simulink model "BoostPFC_ELL437"  (R2022a)
settings: Solver=ode4  StartTime=0.0  StopTime=0.7  FixedStep=1e-7  RelTol=1e-3
undefined symbols (not defined in the file): C, fac, fs_PFC, Gci_inf, Gcv_inf, H, kx, L, R, Rs, vcontrol, Vm, Vref, wLi, wLv
libraries: spsDiodeLib x5, spsSeriesRLCBranchLib x3, spsVoltageMeasurementLib x2, spsACVoltageSourceLib x1, spsCurrentMeasurementLib x1, spsMosfetLib x1, simulink x1, spspowerguiLib x1
settings Model: Creator=Aditya Bhalotia  LastModifiedBy=Aditya Bhalotia
settings DataIOCC: ReturnWorkspaceOutputs=off

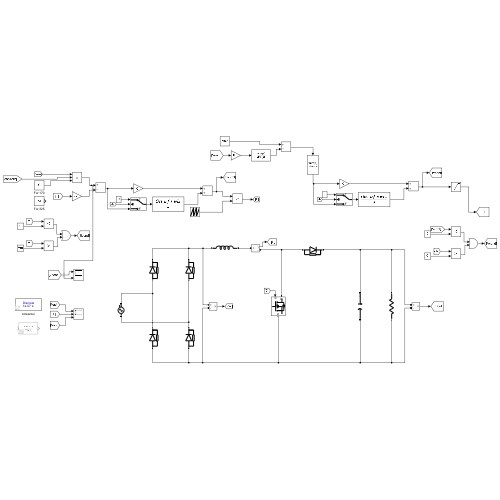
[thumbnail: Simulink's stored preview of the top-level diagram]
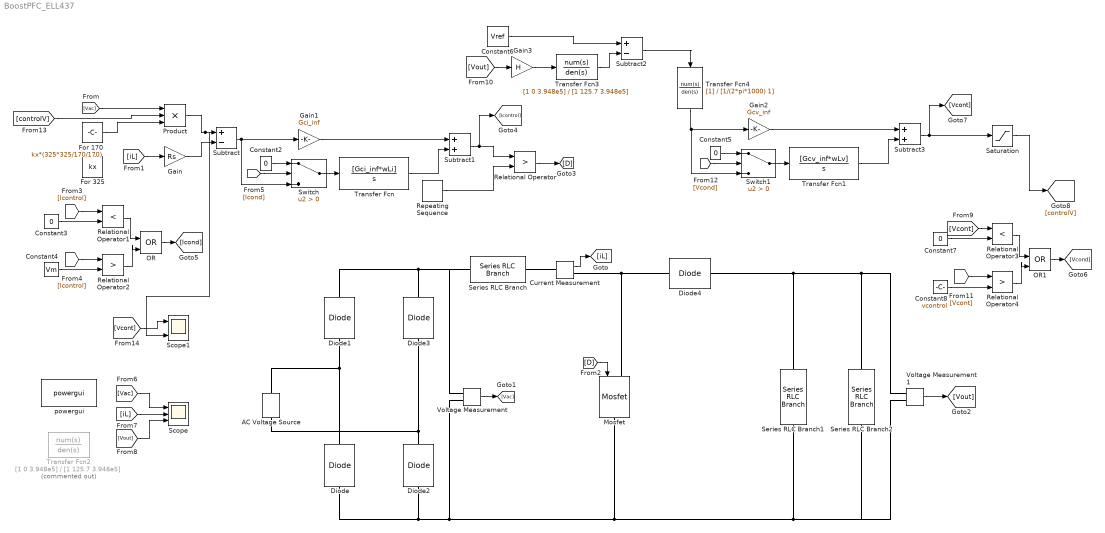
== system BoostPFC_ELL437 ==
  AC Voltage Source : spsACVoltageSourceLib/AC Voltage Source  Amplitude=170  Phase=0  Frequency=fac  SampleTime=0  Measurements=None  BusType=swing  Pref=10e3  Qref=0  Qmin=-inf  Qmax=+inf
  Constant{2..3,5,7} (4 alike) : Constant  Value=0
  Constant4 : Constant  Value=Vm
  Constant6 : Constant  Value=Vref
  Constant8 : Constant  Value=vcontrol
  Current Measurement : spsCurrentMeasurementLib/Current Measurement  PhasorSimulation=off  OutputType=Complex  PSBequivalent=0
  Diode{,1..4} (5 alike) : spsDiodeLib/Diode  Ron=0.001  Lon=0  Vf=0  IC=0  UseSnubber=0  Rs=500  Cs=250e-9  Measurements=off
  For 170 : Constant  Value=kx*(325*325/170/170)
  For 325 : Constant  Value=kx
  Gain : Gain  Gain=Rs
  Gain1 : Gain  Gain=Gci_inf
  Gain2 : Gain  Gain=Gcv_inf
  Gain3 : Gain  Gain=H
  Mosfet : spsMosfetLib/Mosfet  Ron=0.001  Lon=0  Rd=0.001  Vfd=0  IC=0  Rs=1e5  Cs=inf  Measurements=off
  OR : Logic  Operator=OR  IconShape=distinctive  AllPortsSameDT=off  OutDataTypeStr=boolean
  OR1 : Logic  Operator=OR  IconShape=distinctive  AllPortsSameDT=off  OutDataTypeStr=boolean
  Product : Product  Inputs=3
  Relational Operator : RelationalOperator  Operator=>  OutDataTypeStr=boolean  RndMeth=Simplest  InputSameDT=off
  Relational Operator1 : RelationalOperator  Operator=<  OutDataTypeStr=boolean  RndMeth=Simplest  InputSameDT=off
  Relational Operator2 : RelationalOperator  Operator=>  OutDataTypeStr=boolean  RndMeth=Simplest  InputSameDT=off
  Relational Operator3 : RelationalOperator  Operator=<  OutDataTypeStr=boolean  RndMeth=Simplest  InputSameDT=off
  Relational Operator4 : RelationalOperator  Operator=>  OutDataTypeStr=boolean  RndMeth=Simplest  InputSameDT=off
  Repeating Sequence : simulink/Sources/Repeating Sequence  rep_seq_t=[0 1/fs_PFC]  rep_seq_y=[0 Vm]
  Saturation : Saturate  UpperLimit=0.7  LowerLimit=0
  Scope : Scope  NumInputPorts=3
  Scope1 : Scope  NumInputPorts=2
  Series RLC Branch : spsSeriesRLCBranchLib/Series RLC Branch  LConnTagsString=__new0  RConnTagsString=__new0  BranchType=L  Resistance=0  Inductance=L  SetiL0=off  InitialCurrent=0  Capacitance=1e-6  Setx0=off  InitialVoltage=0  Measurements=None
  Series RLC Branch1 : spsSeriesRLCBranchLib/Series RLC Branch  LConnTagsString=__new0  RConnTagsString=__new0  BranchType=C  Resistance=1  Inductance=1e-3  SetiL0=off  InitialCurrent=0  Capacitance=C  Setx0=off  InitialVoltage=0  Measurements=None
  Series RLC Branch2 : spsSeriesRLCBranchLib/Series RLC Branch  LConnTagsString=__new0  RConnTagsString=__new0  BranchType=R  Resistance=R  Inductance=1e-3  SetiL0=off  InitialCurrent=0  Capacitance=1e-6  Setx0=off  InitialVoltage=0  Measurements=None
  Subtract : Sum  Inputs=+-
  Subtract1 : Sum
  Subtract2 : Sum  Inputs=+-
  Subtract3 : Sum
  Switch : Switch  Criteria=u2 > Threshold  SaturateOnIntegerOverflow=off  InputSameDT=off
  Switch1 : Switch  Criteria=u2 > Threshold  SaturateOnIntegerOverflow=off  InputSameDT=off
  Transfer Fcn : TransferFcn  Numerator=[Gci_inf*wLi]  Denominator=[1 0]
  Transfer Fcn1 : TransferFcn  Numerator=[Gcv_inf*wLv]  Denominator=[1 0]
  Transfer Fcn2 : TransferFcn  Commented=on  Numerator=[1 0 3.948e5]  Denominator=[1 125.7 3.948e5]
  Transfer Fcn3 : TransferFcn  Numerator=[1 0 3.948e5]  Denominator=[1 125.7 3.948e5]
  Transfer Fcn4 : TransferFcn  Denominator=[1/(2*pi*1000) 1]
  Voltage Measurement : spsVoltageMeasurementLib/Voltage Measurement  PhasorSimulation=off  OutputType=Complex  PSBequivalent=0
  Voltage Measurement1 : spsVoltageMeasurementLib/Voltage Measurement  PhasorSimulation=off  OutputType=Complex  PSBequivalent=0
  powergui : spspowerguiLib/powergui  Priority=1  SimulationMode=Discrete  SampleTime=1e-7  frequency=60  Iterations=50  frequencyindice=50  Pbase=100e6  ErrMax=1e-4  UnitsV=kV  UnitsW=MW  buscounter=0  FunctionMessages=off  echomessages=off  EnableUseOfTLC=off  CurrentSourceSwitches=off  DisableSnubberDevices=off  DisableRonSwitches=off  DisableVfSwitches=off  DisplayEquations=off  AutomaticDiscreteSolvers=off  SolverType=Tustin/Backward Euler (TBE)  Interpol=off  ExternalGateDelay=off  methode=off  Ts=100  x0status=blocks  SPID=on  SwTol=0  HookPort=off  NonlinearTolerance=1e-4  nMaxIteration=100  ContinueOnMaxIteration=off  RestoreLinks=warning  ResistiveCurrentMeasurement=off  Frange=[0:2:500]  Ylog=off  Xlog=on  ShowGrid=off  save=off  variable=ZData  structure=0  ZoomFFT=off  StartTime=0.0  cycles=1  DisplayStyle=1  fundamental=60  FreqAxis=off  MaxFrequency=1000  frequencyindicesteady=1  RmsSteady=1  display=off
  wires:
  Current Measurement/1 -> [iL]
  Voltage Measurement/1 -> [Vac]
  Voltage Measurement1/1 -> [Vout]
  [Vac] -> Product/1
  [controlV] -> Product/2
  [iL] -> Gain/1
  Product/1 -> Scope1/2, Subtract/1
  Gain/1 -> Subtract/2
  Subtract/1 -> Switch/3, Gain1/1
  Switch/1 -> Transfer Fcn/1
  Constant2/1 -> Switch/1
  Gain1/1 -> Subtract1/1
  Transfer Fcn/1 -> Subtract1/2
  Subtract1/1 -> [Icontrol], Relational Operator/1
  Repeating Sequence/1 -> Relational Operator/2
  Relational Operator/1 -> [D]
  [D] -> Mosfet/1
  [Icontrol] -> Relational Operator1/1
  Constant3/1 -> Relational Operator1/2
  [Icontrol] -> Relational Operator2/1
  Constant4/1 -> Relational Operator2/2
  Relational Operator1/1 -> OR/1
  Relational Operator2/1 -> OR/2
  OR/1 -> [Icond]
  [Icond] -> Switch/2
  [Vac] -> Scope/1
  [iL] -> Scope/2
  [Vout] -> Scope/3
  [Vcond] -> Switch1/2
  Switch1/1 -> Transfer Fcn1/1
  Transfer Fcn1/1 -> Subtract3/2
  Gain2/1 -> Subtract3/1
  Constant5/1 -> Switch1/1
  Subtract2/1 -> Transfer Fcn4/1
  Constant6/1 -> Subtract2/1
  Relational Operator4/1 -> OR1/2
  Relational Operator3/1 -> OR1/1
  Constant8/1 -> Relational Operator4/2
  [Vcont] -> Relational Operator3/1
  [Vcont] -> Relational Operator4/1
  OR1/1 -> [Vcond]
  Constant7/1 -> Relational Operator3/2
  Subtract3/1 -> Saturation/1, [Vcont]
  Saturation/1 -> [controlV]
  [Vout] -> Gain3/1
  Gain3/1 -> Transfer Fcn3/1
  Transfer Fcn4/1 -> Switch1/3, Gain2/1
  [Vcont] -> Scope1/1
  Transfer Fcn3/1 -> Subtract2/2
  For 170/1 -> Product/3
  connections:
  Diode3/RConn1 -- Voltage Measurement/LConn1 -- Series RLC Branch/LConn1 -- Diode1/RConn1
  Diode1/LConn1 -- AC Voltage Source/RConn1 -- Diode/RConn1
  Diode/LConn1 -- Voltage Measurement/LConn2 -- Series RLC Branch2/RConn1 -- Voltage Measurement1/LConn2 -- Series RLC Branch1/RConn1 -- Mosfet/RConn1 -- Diode2/LConn1
  Diode3/LConn1 -- AC Voltage Source/LConn1 -- Diode2/RConn1
  Mosfet/LConn1 -- Diode4/LConn1 -- Current Measurement/RConn1
  Diode4/RConn1 -- Series RLC Branch1/LConn1 -- Series RLC Branch2/LConn1 -- Voltage Measurement1/LConn1
  Series RLC Branch/RConn1 -- Current Measurement/LConn1
